simulink model "testEnvironment"  (R2022b)
settings: Solver=ode4  StartTime=0.0  StopTime=30  FixedStep=0.01  RelTol=1e-3
undefined symbols (not defined in the file or in its folder): bu_ctrlSet, UT, XT
libraries: simulink x4, simulink_extras x3, FMmodelBasic x2, aerolibnav x1, SignalEditorBlockLib x1
settings Model: Creator=Meyer-Brügel  LastModifiedBy=monas
settings SolverCC: AlgebraicLoopSolver=TrustRegion
settings DataIOCC: InitialState=XT  LimitDataPoints=on  SaveFormat=Array  InspectSignalLogs=on  ReturnWorkspaceOutputs=off
settings DataIOCC: ExternalInput=|
  | [r8q_f;r8Th_f;
  | r8uK_f;r8wK_f;r8z_g;r8x_g;r8et;r8gaW;r8gVW;]
settings OptimizationCC: DefaultParameterBehavior=Inlined  ExpressionDepthLimit=2147483647  LifeSpan=inf  SimCompilerOptimization=on
settings DebuggingCC: UnderspecifiedInitializationDetection=Classic  MergeDetectMultiDrivingBlocksExec=none  SolverPrmCheckMsg=warning  MultiTaskDSMMsg=warning  MultiTaskCondExecSysMsg=none  FcnCallInpInsideContextMsg=warning  UnconnectedInputMsg=warning  UnconnectedOutputMsg=warning  UnconnectedLineMsg=warning  StateNameClashWarn=warning  SFUnexpectedBacktrackingDiag=warning  SFNoUnconditionalDefaultTransitionDiag=warning  SFExecutionAtInitializationDiag=none  SFMachineParentedDataDiag=warning  ArithmeticOperatorsInVariantConditions=warning
settings HardwareCC: ProdBitPerLong=64  ProdLargestAtomicFloat=None  ProdHWDeviceType=Intel->x86-64
settings ModelReferenceCC: EnableRefExpFcnMdlSchedulingChecks=on  PropagateSignalLabelsOutOfModel=off
settings SFSimCC: SimUseLocalCustomCode=off  CustomCodeUndefinedFunction=UseInterfaceOnly
settings RTWCC: RTWUseLocalCustomCode=off  DLArmComputeVersion=19.05
settings CodeAppCC: StateflowObjectComments=on
settings GRTTargetCC: TargetLangStandard=C89/C90 (ANSI)  CombineOutputUpdateFcns=off  GRTInterface=on
settings ConfigComp: CovMetricSettings=dw  CovSaveCumulativeToWorkspaceVar=on  CovSaveSingleToWorkspaceVar=on  CovExternalEMLEnable=off  CovSFcnEnable=off

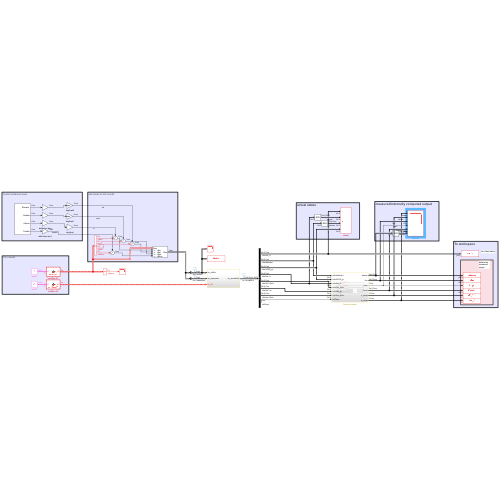
[thumbnail: Simulink's stored preview of the top-level diagram]
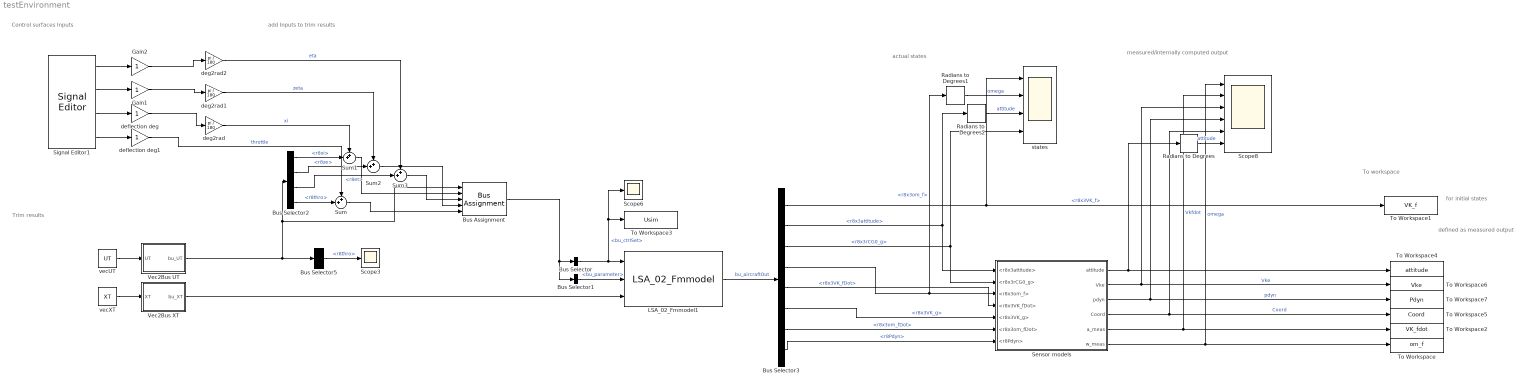
== system testEnvironment ==
  note: measured/internally computed output
  note: defined as measured output
  note: for initial states
  note: To workspace
  note: actual states
  note: add Inputs to trim results
  note: Trim results
  note: Control surfaces Inputs
  Bus Assignment : BusAssignment  AssignedSignals=bu_ctrlSet.r8xi,bu_ctrlSet.r8et,bu_ctrlSet.r8ze,bu_ctrlSet.r8thro
  Bus Selector : BusSelector  OutputSignals=bu_ctrlSet
  Bus Selector1 : BusSelector  OutputSignals=bu_parameter
  Bus Selector2 : BusSelector  OutputSignals=bu_ctrlSet.r8xi,bu_ctrlSet.r8ze,bu_ctrlSet.r8et,bu_ctrlSet.r8thro
  Bus Selector3 : BusSelector  OutputSignals=bu_Xaircraft.bu_XmotionEq.r8x3VK_f,bu_Xaircraft.bu_XmotionEq.r8x3attitude,bu_Xaircraft.bu_XmotionEq.r8x3rCG0_g,bu_Xaircraft.bu_XmotionEq.r8x3om_f,bu_XaircraftDot.bu_XmotionEqDot.r8x3VK_fDot,bu_aircraft.bu_outputVar1.bu_flightPath.r8x3VK_g,bu_XaircraftDot.bu_XmotionEqDot.r8x3om_fDot,bu_aircraft.bu_aero.bu_effFlowARP.r8Pdyn
  Bus Selector5 : BusSelector  OutputSignals=bu_ctrlSet.r8thro
  Gain1 : Gain
  Gain2 : Gain
  LSA_02_Fmmodel1 : FMmodelBasic/LSA_02_Fmmodel  SystemSampleTime=-1  VariantActivationTime=update diagram  Latency=0  AutoFrameSizeCalculation=off
  Radians to Degrees : simulink_extras/Transformations/Radians to Degrees
  Radians to Degrees1 : simulink_extras/Transformations/Radians to Degrees
  Radians to Degrees2 : simulink_extras/Transformations/Radians to Degrees
  Scope3 : Scope
  Scope6 : Scope
  Scope8 : Scope  NumInputPorts=6
  Sensor models : Subsystem
  Signal Editor1 : SignalEditorBlockLib/Signal Editor  FileName=flighttest_maneuvers.mat  ActiveScenario=ElevatorMultistep3211  ActiveSignal=Elevator  IsBus=off  OutputBusObjectStr=Bus: BusObject  SampleTime=0  Interpolate=off  ZeroCross=off  OutputAfterFinalValue=Setting to zero  Unit=inherit  PreserveSignalName=on
  Sum{,1..3} (4 alike) : Sum  Inputs=++|
  To Workspace : ToWorkspace  VariableName=om_f  SaveFormat=Timeseries  SampleTime=-1
  To Workspace1 : ToWorkspace  VariableName=VK_f  SaveFormat=Timeseries  SampleTime=-1
  To Workspace2 : ToWorkspace  VariableName=VK_fdot  SaveFormat=Timeseries  SampleTime=-1
  To Workspace3 : ToWorkspace  VariableName=Usim  SaveFormat=Timeseries  SampleTime=-1
  To Workspace4 : ToWorkspace  VariableName=attitude  SaveFormat=Timeseries  SampleTime=-1
  To Workspace5 : ToWorkspace  VariableName=Coord  SaveFormat=Timeseries  SampleTime=-1
  To Workspace6 : ToWorkspace  VariableName=Vke  SaveFormat=Timeseries  SampleTime=-1
  To Workspace7 : ToWorkspace  VariableName=Pdyn  SaveFormat=Timeseries  SampleTime=-1
  Vec2Bus UT : MATLAB Function  TreatAsAtomicUnit=on
  Vec2Bus XT : MATLAB Function  TreatAsAtomicUnit=on
  deflection deg : Gain
  deflection deg1 : Gain
  deg2rad : Gain  Gain=pi / 180
  deg2rad1 : Gain  Gain=pi / 180
  deg2rad2 : Gain  Gain=pi / 180
  states : Scope  NumInputPorts=4
  vecUT : Constant  Value=UT
  vecXT : Constant  Value=XT
  wires:
  LSA_02_Fmmodel1/1 -> Bus Selector3/1  "bu_aircraftOut"
  vecXT/1 -> Vec2Bus XT/1(XT)
  vecUT/1 -> Vec2Bus UT/1(UT)
  Bus Assignment/1 -> Bus Selector/1, Bus Selector1/1
  Bus Selector/1 -> Scope6/1, To Workspace3/1, LSA_02_Fmmodel1/1  "<bu_ctrlSet>"
  Vec2Bus XT/1(bu_XT) -> LSA_02_Fmmodel1/3
  Bus Selector1/1 -> LSA_02_Fmmodel1/2  "<bu_parameter>"
  Vec2Bus UT/1(bu_UT) -> Bus Selector2/1, Bus Assignment/1, Bus Selector5/1
  Bus Selector2/1 -> Sum1/2  "<r8xi>"
  deflection deg/1 -> deg2rad/1
  deg2rad/1 -> Sum1/1  "xi"
  deg2rad1/1 -> Sum2/1  "zeta"
  deg2rad2/1 -> Sum3/1  "eta"
  Gain2/1 -> deg2rad2/1
  Bus Selector5/1 -> Scope3/1  "<r8thro>"
  Bus Selector2/2 -> Sum2/2  "<r8ze>"
  Bus Selector2/3 -> Sum3/2  "<r8et>"
  Sum1/1 -> Bus Assignment/2
  Sum2/1 -> Bus Assignment/4
  Sum3/1 -> Bus Assignment/3
  Signal Editor1/1 -> Gain2/1
  Bus Selector2/4 -> Sum/2  "<r8thro>"
  Signal Editor1/4 -> deflection deg1/1
  Sum/1 -> Bus Assignment/5
  Gain1/1 -> deg2rad1/1
  Signal Editor1/2 -> Gain1/1
  deflection deg1/1 -> Sum/1  "throttle"
  Signal Editor1/3 -> deflection deg/1
  Bus Selector3/1 -> states/1, To Workspace1/1  "<r8x3VK_f>"
  Bus Selector3/3 -> Sensor models/2(<r8x3rCG0_g>), states/4  "<r8x3rCG0_g>"
  Bus Selector3/2 -> Sensor models/1(<r8x3attitude>), Radians to Degrees2/1  "<r8x3attitude>"
  Radians to Degrees/1 -> Scope8/6  "attitude"
  Bus Selector3/7 -> Sensor models/6(<r8x3om_fDot>)  "<r8x3om_fDot>"
  Radians to Degrees1/1 -> states/2  "omega"
  Sensor models/5(a_meas) -> To Workspace2/1, Scope8/2  "Vkfdot"
  Sensor models/6(w_meas) -> To Workspace/1, Scope8/1  "omega"
  Sensor models/1(attitude) -> To Workspace4/1, Radians to Degrees/1
  Sensor models/3(pdyn) -> To Workspace7/1, Scope8/4  "pdyn"
  Sensor models/4(Coord) -> To Workspace5/1, Scope8/5  "Coord"
  Sensor models/2(Vke) -> To Workspace6/1, Scope8/3  "Vke"
  Bus Selector3/4 -> Radians to Degrees1/1, Sensor models/3(<r8x3om_f>)  "<r8x3om_f>"
  Bus Selector3/5 -> Sensor models/4(<r8x3VK_fDot>)  "<r8x3VK_fDot>"
  Bus Selector3/6 -> Sensor models/5(<r8x3VK_g>)  "<r8x3VK_g>"
  Bus Selector3/8 -> Sensor models/7(<r8Pdyn>)  "<r8Pdyn>"
  Radians to Degrees2/1 -> states/3  "attitude"

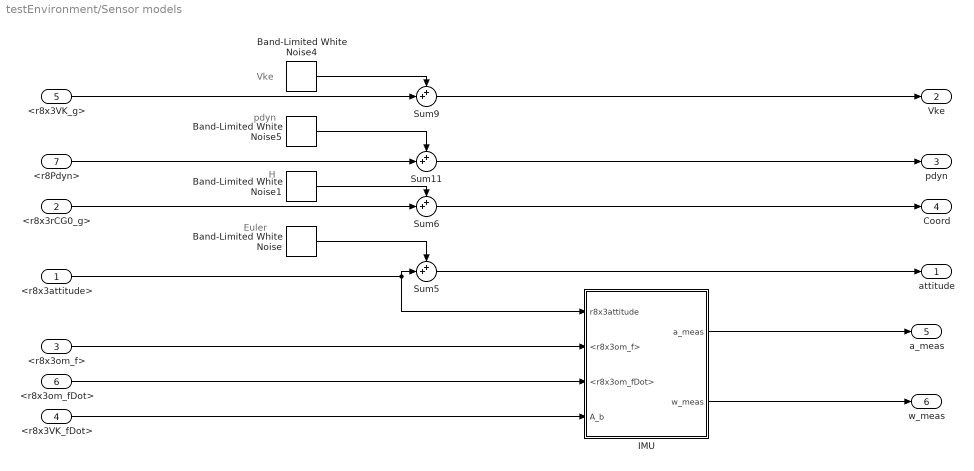
== system testEnvironment/Sensor models ==
  note: Euler
  note: H
  note: pdyn
  note: Vke
  <r8x3attitude> : Inport
  <r8x3rCG0_g> : Inport  Port=2
  <r8x3om_f> : Inport  Port=3
  <r8x3VK_fDot> : Inport  Port=4
  <r8x3VK_g> : Inport  Port=5
  <r8x3om_fDot> : Inport  Port=6
  <r8Pdyn> : Inport  Port=7
  Band-Limited White Noise : simulink/Sources/Band-Limited White Noise  Cov=0.000276*ones(3,1)*0.05  Ts=0.01  seed=[23341;32456;56789]  VectorParams1D=off
  Band-Limited White Noise1 : simulink/Sources/Band-Limited White Noise  Cov=0.0756*ones(3,1)*1  Ts=0.01  seed=[20341;32411;53489]  VectorParams1D=off
  Band-Limited White Noise4 : simulink/Sources/Band-Limited White Noise  Cov=ones(3,1)*0.0037*1  Ts=0.01  seed=[203241;3245611;5348549]  VectorParams1D=off
  Band-Limited White Noise5 : simulink/Sources/Band-Limited White Noise  Cov=3.92*1  Ts=0.01  seed=[25341]  VectorParams1D=off
  IMU : Subsystem
  Sum{5..6,9,11} (4 alike) : Sum  Inputs=++|
  attitude : Outport
  Vke : Outport  Port=2
  pdyn : Outport  Port=3
  Coord : Outport  Port=4
  a_meas : Outport  Port=5
  w_meas : Outport  Port=6
  wires:
  Band-Limited White Noise1/1 -> Sum6/1
  <r8x3VK_g>/1 -> Sum9/2
  Band-Limited White Noise4/1 -> Sum9/1
  <r8Pdyn>/1 -> Sum11/2
  <r8x3attitude>/1 -> Sum5/2, IMU/1(r8x3attitude)
  Sum6/1 -> Coord/1
  Sum11/1 -> pdyn/1
  Band-Limited White Noise/1 -> Sum5/1
  Band-Limited White Noise5/1 -> Sum11/1
  <r8x3om_fDot>/1 -> IMU/3(<r8x3om_fDot>)
  Sum5/1 -> attitude/1
  Sum9/1 -> Vke/1
  <r8x3VK_fDot>/1 -> IMU/4(A_b)
  <r8x3rCG0_g>/1 -> Sum6/2
  <r8x3om_f>/1 -> IMU/2(<r8x3om_f>)
  IMU/2(w_meas) -> w_meas/1
  IMU/1(a_meas) -> a_meas/1

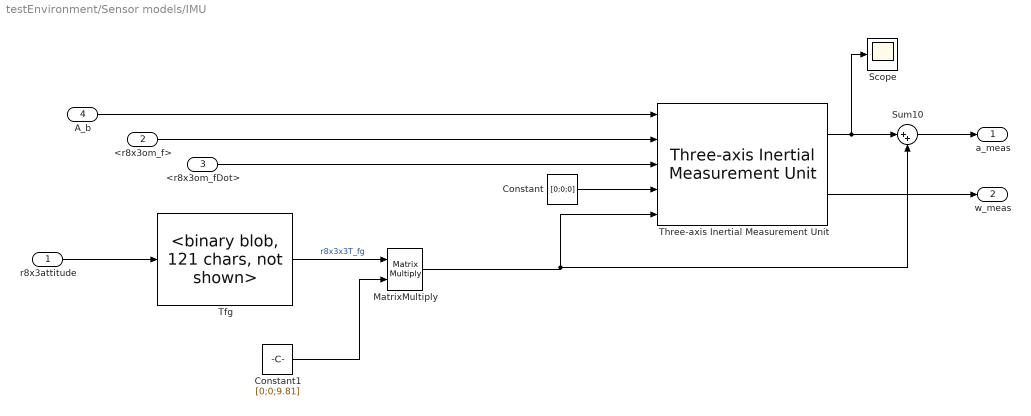
== system testEnvironment/Sensor models/IMU ==
  r8x3attitude : Inport
  <r8x3om_f> : Inport  Port=2
  <r8x3om_fDot> : Inport  Port=3
  A_b : Inport  Port=4
  Constant : Constant  Value=[0;0;0]
  Constant1 : Constant  Value=[0;0;9.81]
  MatrixMultiply : Product  Multiplication=Matrix(*)
  Scope : Scope
  Sum10 : Sum  Inputs=|++
  Tfg : FMmodelBasic/LSA_02_Fmmodel/aircraft/2_output_variables_part1/22_coordinate_transformations/221_geodetic_to_bodyfixed/Tfg  SystemSampleTime=-1  VariantActivationTime=update diagram  Latency=0  AutoFrameSizeCalculation=off
  Three-axis Inertial Measurement Unit : aerolibnav/Three-axis Inertial Measurement Unit  units=Metric (MKS)  imu=[0 0 0]  i_Ts=0  dtype_a=on  w_a=120  z_a=0.7  a_sf_cc=[1 0 0; 0 1 0; 0 0 1]  a_bias=[0 0 0]  a_sat=[-16 -16 -16 16 16 16]*9.81  dtype_g=on  w_g=120  z_g=0.70  g_sf_cc=[1 0 0; 0 1 0; 0 0 1]  g_bias=[0 0 0]  g_sens=[0 0 0]  g_sat=[-2000 -2000 -2000 2000 2000 2000]  i_rand=on  i_seeds=[23093 23094 23095 23096 23097 23098]  i_pow=[0.000147 0.000147 0.000147 0.0000244 0.0000244 0.0000244]
  a_meas : Outport
  w_meas : Outport  Port=2
  wires:
  MatrixMultiply/1 -> Three-axis Inertial Measurement Unit/5, Sum10/2
  Constant/1 -> Three-axis Inertial Measurement Unit/4
  A_b/1 -> Three-axis Inertial Measurement Unit/1
  r8x3attitude/1 -> Tfg/1
  Three-axis Inertial Measurement Unit/1 -> Scope/1, Sum10/1
  <r8x3om_fDot>/1 -> Three-axis Inertial Measurement Unit/3
  Tfg/1 -> MatrixMultiply/1  "r8x3x3T_fg"
  Constant1/1 -> MatrixMultiply/2
  <r8x3om_f>/1 -> Three-axis Inertial Measurement Unit/2
  Three-axis Inertial Measurement Unit/2 -> w_meas/1
  Sum10/1 -> a_meas/1

== matlab function testEnvironment/Vec2Bus XT ==
  data: XT input; bu_XT output Bus: bu_XT
function bu_XT = vec2busXT(XT)

bu_XT.bu_XmotionEqT.r8x3om_fT =XT(1:3);
bu_XT.bu_XmotionEqT.r8x3attitudeT =XT(4:6);
bu_XT.bu_XmotionEqT.r8x3VK_fT =XT(7:9);
bu_XT.bu_XmotionEqT.r8x3rCG0_gT =XT(10:12);

end

== matlab function testEnvironment/Vec2Bus UT ==
  data: UT input; bu_UT output Bus: bu_UT
function bu_UT = vec2busUT(UT)

bu_UT.bu_ctrlSet.r8xi =UT(1:1);
bu_UT.bu_ctrlSet.r8et =UT(2:2);
bu_UT.bu_ctrlSet.r8ze =UT(3:3);
bu_UT.bu_ctrlSet.r8thro =UT(4:4);
bu_UT.bu_ctrlSet.r8ets =UT(5:5);
bu_UT.bu_ctrlSet.r8etk =UT(6:6);
bu_UT.bu_ctrlSet.r8gearDwn =UT(7:7);
bu_UT.bu_ctrlSet.r8omProp_c =UT(8:8);
bu_UT.bu_ctrlSet.r8etTrm =UT(9:9);
bu_UT.bu_parameter.bu_windPar.r8VW =UT(10:10);
bu_UT.bu_parameter.bu_windPar.r8gaW =UT(11:11);
bu_UT.bu_parameter.bu_windPar.r8ChW =UT(12:12);
bu_UT.bu_parameter.bu_inertPar.r8IOEWxx_f =UT(13:13);
bu_UT.bu_parameter.bu_inertPar.r8IOEWyy_f =UT(14:14);
bu_UT.bu_parameter.bu_inertPar.r8IOEWzz_f =UT(15:15);
bu_UT.bu_parameter.bu_inertPar.r8IOEWxy_f =UT(16:16);
bu_UT.bu_parameter.bu_inertPar.r8IOEWxz_f =UT(17:17);
bu_UT.bu_parameter.bu_inertPar.r8IOEWyz_f =UT(18:18);
bu_UT.bu_parameter.bu_inertPar.r8mOEW =UT(19:19);

% funtion 2 create like this save corresponding text file 
% UT(1)=double(bu_UT.bu_ctrlSet.r8xi);

end
